simulink model "qbmove_simulink_example"  (Simulink 7.9)
settings: Solver=ode3  StartTime=0.0  StopTime=inf  FixedStep=1e-2  RelTol=1e-3
libraries: simulink x2, qbmove_library x1
settings Model: Creator=laurentio  LastModifiedBy=laurentio

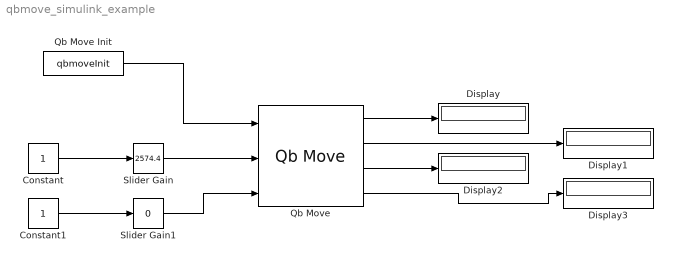
== system qbmove_simulink_example ==
  Constant : Constant
  Constant1 : Constant
  Display{,1..3} (4 alike) : Display
  Qb Move : qbmove_library/Qb Move  ID=65  ACTIVE_COMM_DIRECTIONS=Both  CONTROL_MODE=Prime Movers Positions  DAISY_CHAINING=off  MAX_ANG=0  SW_LIMIT=inf  OFFSET=0
  Qb Move Init : S-Function  AncestorBlock=qbmove_library/Qb Move Init  FunctionName=qbmoveInit  Parameters=double(NUMBER_OF_COM), 115200  EnableBusSupport=off  mask(qb Init - ISS){NUMBER_OF_COM='/dev/tty.usbserial-DAWQMBM3'}
      mask prompts: NUMBER_OF_COM "USB-ISS Virtual COM port number"
      mask help: qb devices initialization block.
      mask TabNameString: Serial Port Configuration
      mask Display:
      | % image( imread('bridge.jpg') )
      | port_label( 'output', 1, 'handle' );
  Slider Gain : simulink/Math Operations/Slider Gain  low=-100000  gain=2574.4  high=100000
  Slider Gain1 : simulink/Math Operations/Slider Gain  low=-10000  gain=0  high=10000
  wires:
  Qb Move Init/1 -> Qb Move/1
  Constant/1 -> Slider Gain/1
  Slider Gain/1 -> Qb Move/2
  Constant1/1 -> Slider Gain1/1
  Slider Gain1/1 -> Qb Move/3
  Qb Move/1 -> Display/1
  Qb Move/2 -> Display1/1
  Qb Move/3 -> Display2/1
  Qb Move/4 -> Display3/1
